simulink model "chap3_sim"  (R2025b)
settings: Solver=ode45  StartTime=0.0  StopTime=20  MaxStep=0.05  RelTol=1e-3
settings Model: Creator=ASUS  LastModifiedBy=ASUS

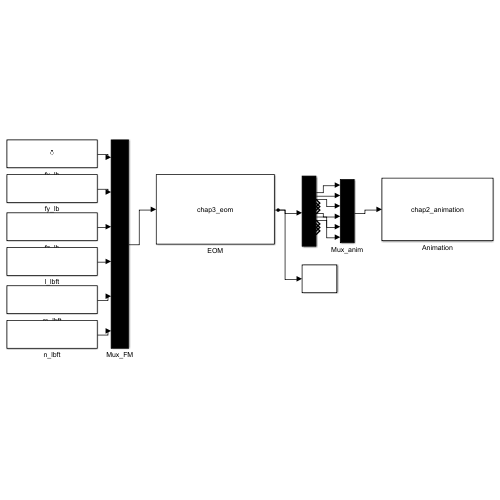
[thumbnail: Simulink's stored preview of the top-level diagram]
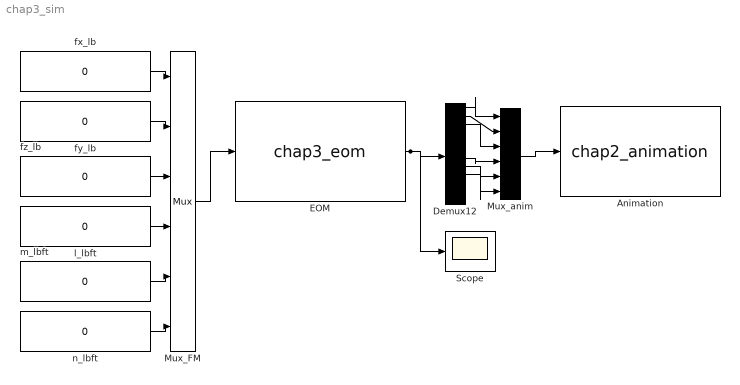
== system chap3_sim ==
  Animation : M-S-Function  FunctionName=chap2_animation  Parameters=1
  Demux12 : Demux  Outputs=12
  EOM : M-S-Function  FunctionName=chap3_eom  Parameters=1212.16,25000,122200,139800,2200, 0,0,-300, 0,0,0, 0,0,0, 0,0,0
  Mux_FM : Mux  Inputs=6
  Mux_anim : Mux  Inputs=6
  Scope : Scope
  fx_lb : Constant  Value=0  OutDataTypeStr=double
  fy_lb : Constant  Value=0  OutDataTypeStr=double
  fz_lb : Constant  Value=0  OutDataTypeStr=double
  l_lbft : Constant  Value=0  OutDataTypeStr=double
  m_lbft : Constant  Value=0  OutDataTypeStr=double
  n_lbft : Constant  Value=0  OutDataTypeStr=double
  wires:
  fx_lb/1 -> Mux_FM/1
  fy_lb/1 -> Mux_FM/2
  fz_lb/1 -> Mux_FM/3
  l_lbft/1 -> Mux_FM/4
  m_lbft/1 -> Mux_FM/5
  n_lbft/1 -> Mux_FM/6
  Mux_FM/1 -> EOM/1
  EOM/1 -> Demux12/1, Scope/1
  Demux12/1 -> Mux_anim/1
  Demux12/2 -> Mux_anim/2
  Demux12/3 -> Mux_anim/3
  Demux12/7 -> Mux_anim/4
  Demux12/8 -> Mux_anim/5
  Demux12/9 -> Mux_anim/6
  Mux_anim/1 -> Animation/1
